simulink library "MotorModelDiscreteSL"  (R2016b)
settings: Solver=VariableStepAuto  StartTime=0.0  StopTime=10.0  RelTol=1e-3
undefined symbols (not defined in the file): CAL_B_NmPerW, CAL_flux_e, CAL_flux_t, CAL_Inertia_J, CAL_Re_ohm, CAL_SAMPLE_TIME, CAL_SimInduct_H
settings Model: Creator=oelkawok  LastModifiedBy=oelkawok

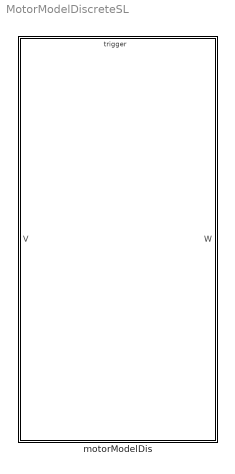
== system MotorModelDiscreteSL ==
  motorModelDis : Subsystem

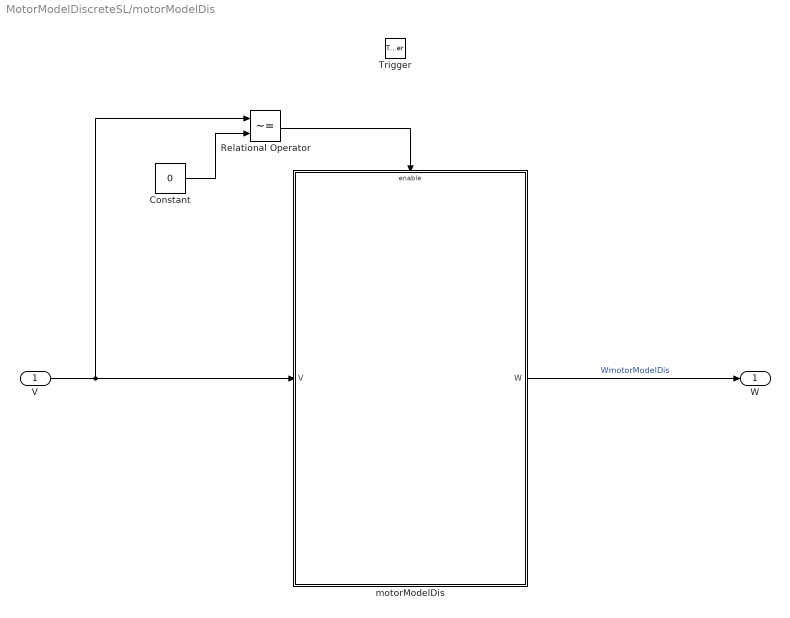
== system MotorModelDiscreteSL/motorModelDis ==
  V : Inport
  Trigger : TriggerPort  TriggerType=function-call  VariantControl=Variant  PortDimensions=1
  Constant : Constant  Value=0
  Relational Operator : RelationalOperator  Operator=~=  OutDataTypeStr=boolean  RndMeth=Simplest
  motorModelDis : Subsystem
  W : Outport
  wires:
  Relational Operator/1 -> motorModelDis/Enable
  Constant/1 -> Relational Operator/2
  motorModelDis/1(W) -> W/1  "WmotorModelDis"
  V/1 -> motorModelDis/1(V), Relational Operator/1

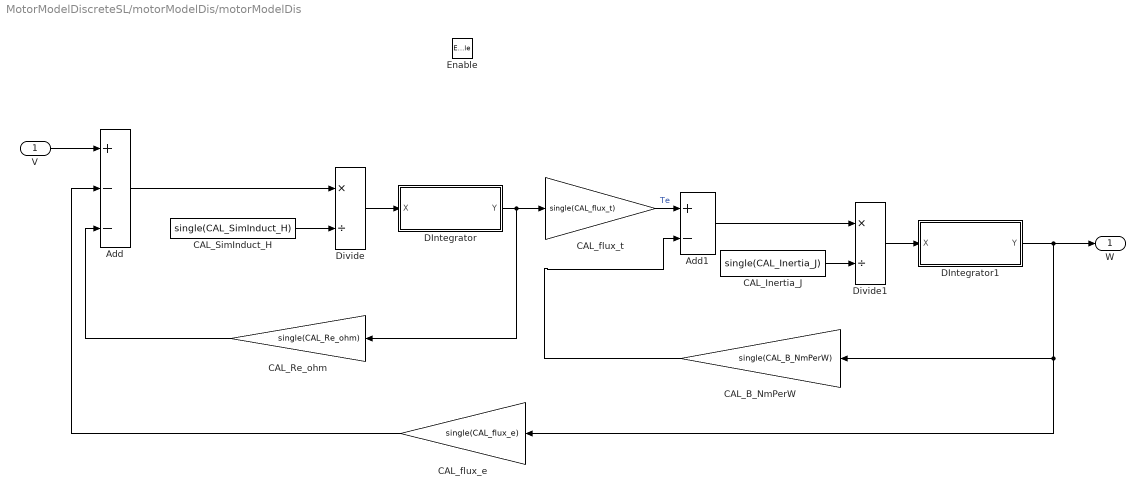
== system MotorModelDiscreteSL/motorModelDis/motorModelDis ==
  V : Inport
  Enable : EnablePort  StatesWhenEnabling=reset
  Add : Sum  Inputs=+--
  Add1 : Sum  Inputs=+-
  CAL_B_NmPerW : Gain  Gain=single(CAL_B_NmPerW)
  CAL_Inertia_J : Constant  Value=single(CAL_Inertia_J)
  CAL_Re_ohm : Gain  Gain=single(CAL_Re_ohm)
  CAL_SimInduct_H : Constant  Value=single(CAL_SimInduct_H)
  CAL_flux_e : Gain  Gain=single(CAL_flux_e)
  CAL_flux_t : Gain  Gain=single(CAL_flux_t)
  DIntegrator : Subsystem
  DIntegrator1 : Subsystem
  Divide : Product  Inputs=*/
  Divide1 : Product  Inputs=*/
  W : Outport  OutputWhenDisabled=reset  InitialOutput=0
  wires:
  Add/1 -> Divide/1
  CAL_B_NmPerW/1 -> Add1/2
  Add1/1 -> Divide1/1
  CAL_flux_e/1 -> Add/2
  CAL_flux_t/1 -> Add1/1  "Te"
  CAL_Inertia_J/1 -> Divide1/2
  CAL_SimInduct_H/1 -> Divide/2
  CAL_Re_ohm/1 -> Add/3
  V/1 -> Add/1
  Divide/1 -> DIntegrator/1(X)
  DIntegrator/1(Y) -> CAL_Re_ohm/1, CAL_flux_t/1
  Divide1/1 -> DIntegrator1/1(X)
  DIntegrator1/1(Y) -> CAL_flux_e/1, CAL_B_NmPerW/1, W/1

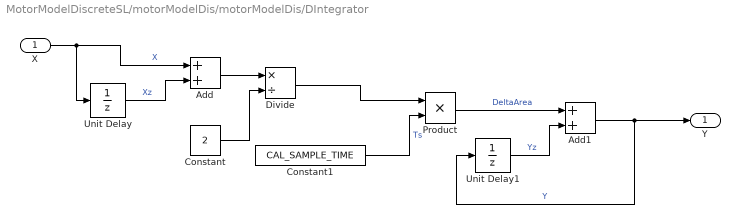
== system MotorModelDiscreteSL/motorModelDis/motorModelDis/DIntegrator ==
  X : Inport
  Add : Sum
  Add1 : Sum
  Constant : Constant  Value=2
  Constant1 : Constant  Value=CAL_SAMPLE_TIME
  Divide : Product  Inputs=*/
  Product : Product
  Unit Delay : UnitDelay  SampleTime=-1
  Unit Delay1 : UnitDelay  SampleTime=-1
  Y : Outport
  wires:
  Unit Delay/1 -> Add/2  "Xz"
  X/1 -> Unit Delay/1, Add/1  "X"
  Add/1 -> Divide/1
  Constant/1 -> Divide/2
  Constant1/1 -> Product/2  "Ts"
  Divide/1 -> Product/1
  Product/1 -> Add1/1  "DeltaArea"
  Add1/1 -> Unit Delay1/1, Y/1  "Y"
  Unit Delay1/1 -> Add1/2  "Yz"

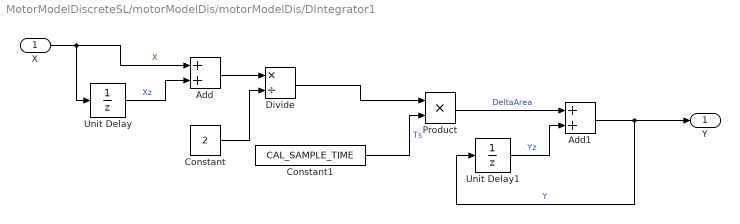
== system MotorModelDiscreteSL/motorModelDis/motorModelDis/DIntegrator1 ==
  X : Inport
  Add : Sum
  Add1 : Sum
  Constant : Constant  Value=2
  Constant1 : Constant  Value=CAL_SAMPLE_TIME
  Divide : Product  Inputs=*/
  Product : Product
  Unit Delay : UnitDelay  SampleTime=-1
  Unit Delay1 : UnitDelay  SampleTime=-1
  Y : Outport
  wires:
  Unit Delay1/1 -> Add1/2  "Yz"
  Add1/1 -> Y/1, Unit Delay1/1  "Y"
  Product/1 -> Add1/1  "DeltaArea"
  Divide/1 -> Product/1
  Constant1/1 -> Product/2  "Ts"
  Constant/1 -> Divide/2
  Add/1 -> Divide/1
  X/1 -> Add/1, Unit Delay/1  "X"
  Unit Delay/1 -> Add/2  "Xz"
